simulink model "weightlose4"  (R2021b)
settings: Solver=VariableStepAuto  StartTime=0.0  StopTime=500  RelTol=1e-3
libraries: cstblocks x1
settings Model: Creator=DELL  LastModifiedBy=DELL

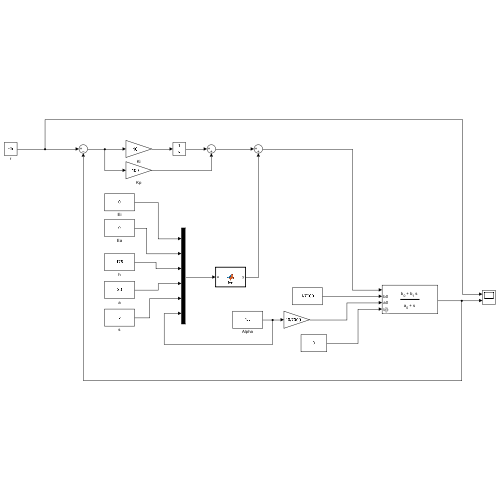
[thumbnail: Simulink's stored preview of the top-level diagram]
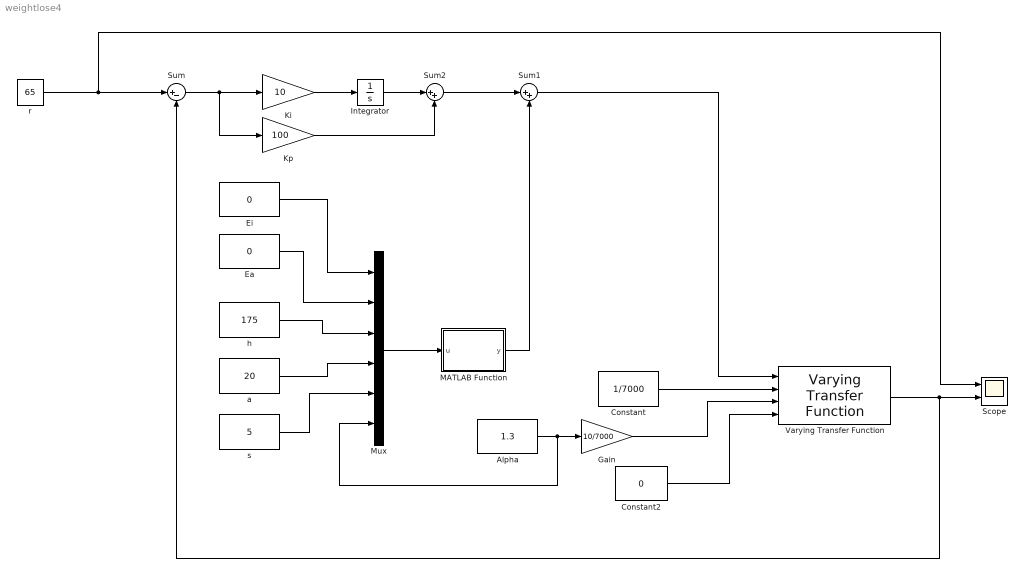
== system weightlose4 ==
  Alpha : Constant  Value=1.3
  Constant : Constant  Value=1/7000
  Constant2 : Constant  Value=0
  Ea : Constant  Value=0
  Ei : Constant  Value=0
  Gain : Gain  Gain=10/7000
  Integrator : Integrator
  Ki : Gain  Gain=10
  Kp : Gain  Gain=100
  MATLAB Function : MATLAB Function  TreatAsAtomicUnit=on
  Mux : Mux  Inputs=6
  Scope : Scope  NumInputPorts=2
  Sum : Sum  Inputs=|+-
  Sum1 : Sum  Inputs=|++
  Sum2 : Sum  Inputs=|++
  Varying Transfer Function : cstblocks/Linear Parameter Varying/Varying Transfer Function  N=1
      link override Integrator1: InitialCondition=70
  a : Constant  Value=20
  h : Constant  Value=175
  r : Constant  Value=65
  s : Constant  Value=5
  wires:
  r/1 -> Scope/1, Sum/1
  Varying Transfer Function/1 -> Sum/2, Scope/2
  Constant/1 -> Varying Transfer Function/2
  MATLAB Function/1(y) -> Sum1/2
  Sum/1 -> Kp/1, Ki/1
  Sum1/1 -> Varying Transfer Function/1
  Ki/1 -> Integrator/1
  Ei/1 -> Mux/1
  Gain/1 -> Varying Transfer Function/3
  s/1 -> Mux/5
  Mux/1 -> MATLAB Function/1(u)
  Constant2/1 -> Varying Transfer Function/4
  Alpha/1 -> Mux/6, Gain/1
  a/1 -> Mux/4
  h/1 -> Mux/3
  Ea/1 -> Mux/2
  Kp/1 -> Sum2/2
  Integrator/1 -> Sum2/1
  Sum2/1 -> Sum1/1

== matlab function weightlose4/MATLAB Function ==
  data: u input; y output
function y = fcn(u)

y = u(1)-u(2)-u(6)*(6.25*u(3)-5*u(4)+u(5));
